simulink model "single_phase_bridge_Rectifier_R"  (R2015a)
settings: Solver=ode45  StartTime=0.0  StopTime=0.05  RelTol=1e-3
libraries: powerlib x10
settings Model: Creator=HP  LastModifiedBy=HP

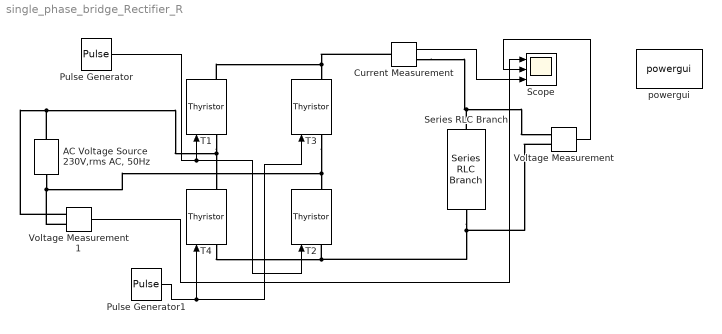
== system single_phase_bridge_Rectifier_R ==
  "AC Voltage Source 230V,rms AC, 50Hz" : powerlib/Electrical Sources/AC Voltage Source  Amplitude=325  Phase=0  Frequency=50  SampleTime=0  Measurements=None
  Current Measurement : powerlib/Measurements/Current Measurement  PhasorSimulation=off  OutputType=Complex  PSBequivalent=0
  Pulse Generator : DiscretePulseGenerator  PulseType=Time based  Amplitude=50  Period=1/50  PulseWidth=5  PhaseDelay=30/(50*360)
  Pulse Generator1 : DiscretePulseGenerator  PulseType=Time based  Amplitude=50  Period=1/50  PulseWidth=5  PhaseDelay=210/(50*360)
  Scope : Scope  NumInputPorts=3
      settings: YMin=-600~-600~-600  YMax=600~600~600
  Series RLC Branch : powerlib/Elements/Series RLC Branch  LConnTagsString=__new0  RConnTagsString=__new0  BranchType=RL  Resistance=1  Inductance=1e-3  SetiL0=off  InitialCurrent=0  Capacitance=1e-6  Setx0=off  InitialVoltage=0  Measurements=None
  T{1..4} (4 alike) : powerlib/Power Electronics/Thyristor  Ron=0.001  Lon=0  Vf=0.8  IC=0  Rs=500  Cs=250e-9  Measurements=on
  Voltage Measurement : powerlib/Measurements/Voltage Measurement  PhasorSimulation=off  OutputType=Complex  PSBequivalent=0
  Voltage Measurement1 : powerlib/Measurements/Voltage Measurement  PhasorSimulation=off  OutputType=Complex  PSBequivalent=0
  powergui : powerlib/powergui  Priority=1  SimulationMode=Continuous  SolverType=Tustin/Backward Euler (TBE)  SampleTime=50e-6  frequency=60  SPID=off  DisableSnubberDevices=off  DisableRonSwitches=off  DisableVfSwitches=off  SwTol=0  DisplayEquations=off  Interpol=off  methode=off  Ts=100  FunctionMessages=off  echomessages=off  HookPort=off  EnableUseOfTLC=off  x0status=blocks  frequencyindice=50  Pbase=100e6  ErrMax=1e-4  Iterations=50  UnitsV=kV  UnitsW=MW  buscounter=0  RestoreLinks=warning  ResistiveCurrentMeasurement=off  Frange=[0:2:500]  Ylog=off  Xlog=on  ShowGrid=off  save=off  variable=ZData  structure=0  ZoomFFT=off  StartTime=0.0  cycles=1  DisplayStyle=1  fundamental=60  FreqAxis=off  MaxFrequency=1000  frequencyindicesteady=1  RmsSteady=1  display=off
  wires:
  Voltage Measurement1/1 -> Scope/1
  Voltage Measurement/1 -> Scope/2
  Pulse Generator1/1 -> T3/1, T4/1
  Pulse Generator/1 -> T2/1, T1/1
  Current Measurement/1 -> Scope/3
  connections:
  T1/LConn1 -- "AC Voltage Source 230V,rms AC, 50Hz"/RConn1 -- Voltage Measurement1/LConn1 -- T4/RConn1
  T3/LConn1 -- Voltage Measurement1/LConn2 -- "AC Voltage Source 230V,rms AC, 50Hz"/LConn1 -- T2/RConn1
  Current Measurement/RConn1 -- Series RLC Branch/LConn1 -- Voltage Measurement/LConn1
  T4/LConn1 -- Voltage Measurement/LConn2 -- Series RLC Branch/RConn1 -- T2/LConn1
  T1/RConn1 -- Current Measurement/LConn1 -- T3/RConn1
